simulink library "Pump_Additional"  (R2018b)
settings: Solver=ode45  StartTime=0.0  StopTime=10.0  RelTol=1e-3  EnableMultiTasking=on
undefined symbols (not defined in the file): DiameterLastPiece, DPConstant, DPLinear, DPQuadratic, ID, path_carnot, Pressure, Temperature
libraries: carnot x3
settings Model: Creator=Hafner  LastModifiedBy=drhf
settings DataIOCC: LimitDataPoints=on  SaveFormat=Array  SignalLoggingSaveFormat=ModelDataLogs
settings OptimizationCC: ExpressionDepthLimit=2147483647  LifeSpan=inf
settings DebuggingCC: UnderspecifiedInitializationDetection=Classic  MergeDetectMultiDrivingBlocksExec=none  SolverPrmCheckMsg=warning  FcnCallInpInsideContextMsg=warning  StateNameClashWarn=warning  SFUnexpectedBacktrackingDiag=warning  SFNoUnconditionalDefaultTransitionDiag=warning  SFExecutionAtInitializationDiag=none
settings HardwareCC: ProdBitPerPointer=32  ProdBitPerSizeT=32  ProdBitPerPtrDiffT=32  ProdLargestAtomicFloat=None  ProdIntDivRoundTo=Undefined  ProdEndianess=Unspecified  ProdWordSize=32  ProdHWDeviceType=32-bit Generic
settings ModelReferenceCC: PropagateSignalLabelsOutOfModel=off
settings SFSimCC: SimUseLocalCustomCode=off
settings RTWCC: RTWUseLocalCustomCode=off
settings CodeAppCC: StateflowObjectComments=on
settings GRTTargetCC: TargetLangStandard=C89/C90 (ANSI)  GeneratePreprocessorConditionals=Disable all  CombineOutputUpdateFcns=off  GRTInterface=on
settings ConfigComp: CovMetricSettings=dw  CovHtmlReporting=on  CovSaveCumulativeToWorkspaceVar=on  CovSaveSingleToWorkspaceVar=on  CovExternalEMLEnable=off

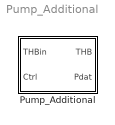
== system Pump_Additional ==
  Pump_Additional : Subsystem  mask(Pump Additional){Tini=20, PathName=fullfile(path_carnot('libsl'), 'Hydraulics', 'Pump_Main', 'parameter_set'), FileName='Pump6m.mat', userPath=off, userParam=off, a0=60000, a1=-43200, a2=0, dia=0.025, UA=1, mcp=4182, e0=50, e1=28.8, e2=-10.368}
      mask prompts: Tini "Ambient temperature for losses and initial temperture in °C"; PathName "Path"; FileName "Parameter set"; userPath "Edit path and name of parameter set"; userParam "User defined parameters"; a0 "a0: pump head in [Pa] (pressure increase at zero flow)"; a1 "a1: pump characteristic linear coefficient [Pa*s/kg]"; a2 "a2: pump characteristic quadratic coefficient [Pa*(s/kg)²]"; dia "Diameter at in- and outlet [m]"; UA "UA: thermal loss coefficient in W/K"; mcp "mcp: thermal capacity of the node in J/K"; e0 "e0: constant coefficient in W"; e1 "e1: linear coefficient in W*s/kg"; e2 "e2: quadratic coefficient in W*(s/kg)²"
      mask help:
      | This is an additional pump in a circuit. Every circuit must have exactly ONE 'Pump_Main'. It may have several 'Pump_Additional' blocks. The pump adds dp_pump to the pressure drop of the circuit dp_circuit:
      |     dp_circuit = c + l*mdot + q*(mdot)²
      |     dp_pump_ = a0*Ctrl + a1*mdot +a2*(mdot)²
      |     dp_total = dp_pump - dp_circuit
      |     p1 = system_pressure + (a0*Ctrl - c) + (a1 - l) * mdot + (a2-q)*(mdot)²
      | with
      |   Ctrl : Control signal input [0..1]
      | Note: Pump_Additional uses the parameters sets as Pump_Main.
      mask init:
      | % callback to set parameters of model
      | [ok, param] = CarnotCallbacks_PumpAdditional('SetParameters',gcbh,PathName,FileName);
      mask Help: web(fullfile(path_carnot('help'),'Pump_Main.html'),'-helpbrowser')
      mask TypeOptions Tini: ThermalNodeTHB/Tini
      mask Callback userPath: [ok, param] = CarnotCallbacks_PumpAdditional('UserEdit',gcbh);
      mask Callback userParam: [ok, param] = CarnotCallbacks_PumpAdditional('UserEdit',gcbh);
      mask TypeOptions a0: PumpHead/Gain
      mask TypeOptions a1: PumpLinear/Value
      mask TypeOptions a2: PumpQuadratic/Value
      mask TypeOptions dia: dia/Value
      mask TypeOptions UA: ThermalNodeTHB/UA
      mask TypeOptions mcp: ThermalNodeTHB/mcp
      mask TypeOptions e0: ElectricConsumptionPump/e0
      mask TypeOptions e1: ElectricConsumptionPump/e1
      mask TypeOptions e2: ElectricConsumptionPump/e2
      mask DialogControl ParameterGroupFile Prompt: Picking a parameter set
      mask DialogControl Control1 Prompt: Carnot public data
      mask DialogControl Control1 Callback: [ok, file] = CarnotCallbacks_PumpAdditional('GetFilename',gcbh,'public');
      mask DialogControl Control3 Prompt: Carnot internal data
      mask DialogControl Control3 Callback: [ok, file] = CarnotCallbacks_PumpAdditional('GetFilename',gcbh,'internal');
      mask DialogControl Control4 Prompt: Selected path
      mask DialogControl Control4 Callback: [ok, file] = CarnotCallbacks_PumpAdditional('GetFilename',gcbh,'selected');
      mask DialogControl PrameterGroupUser Prompt: Parameter Values
      mask DialogControl Container9 Prompt: Hydraulic
      mask DialogControl Container7 Prompt: Thermal
      mask DialogControl Control9 Prompt: Thermal node for temperature:  mcp * dTnode/dt = UA*(Tamb-Tnode) + mdot*cp_in*(Tin-Tnode)
      mask DialogControl Container12 Prompt: Electric
      mask DialogControl Control7 Prompt: Power consumption  Pel = e0 + e1*mdot + e2*mdot²
      mask DialogControl Control5 Prompt: Save in Carnot internal data
      mask DialogControl Control5 Callback: [ok, param] = CarnotCallbacks_PumpAdditional('SaveFilename',gcbh,'internal','B');
      mask DialogControl Control6 Prompt: Save in selected path
      mask DialogControl Control6 Callback: [ok, param] = CarnotCallbacks_PumpAdditional('SaveFilename',gcbh,'selected','B');
      mask Display:
      | % user defined picture file
      | picfile = fullfile(path_carnot('intlibsl'), ...
      |         'Hydraulics', 'Pump_Additional', 'PumpAdditional.jpg');
      | 
      | pic = false;
      | if ~BlockIsInCarnotLibrary    % if not located in library any more
      |     if exist(picfile,'file') % show internal picture if defined
      |         image(imread(picfile), [0.2, 0, 0.6, 1])
      |         set_param(gcb, 'BackgroundColor', 'White')
      |         pic = true;
      |     end
      | end
      | if ~pic    % show public picture
      |     set_param(gcb, 'BackgroundColor', 'green')
      |     plot(0,0,1,1,[40,70,40,30,30,40,60,70,70,60,40]/100, ...
      |         [70,50,30,40,60,70,70,60,40,30,30]/100)
      |     disp('add')
      | end

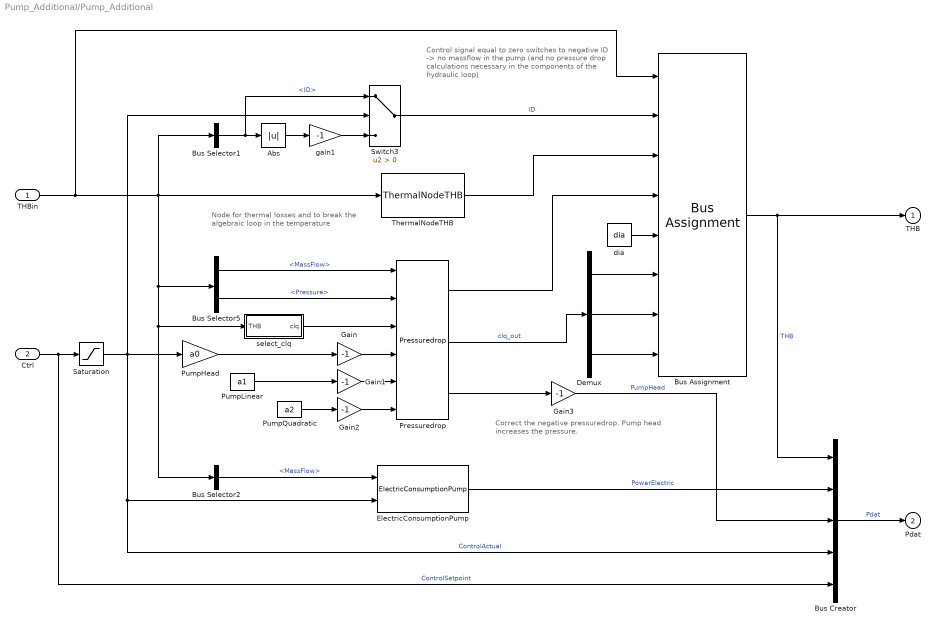
== system Pump_Additional/Pump_Additional ==
  note: Node for thermal losses and to break
      | the algebraic loop in the temperature
  note: Control signal equal to zero switches
      | to negative ID -> no massflow in the
      | pump (and no pressure drop calculations
      | necessary in the components of the
      | hydraulic loop)
  note: Correct the negative pressuredrop.
      | Pump head increases the pressure.
  THBin : Inport
  Ctrl : Inport  Port=2
  Abs : Abs
  Bus Assignment : BusAssignment  AssignedSignals=ID,Temperature,Pressure,DiameterLastPiece,DPConstant,DPLinear,DPQuadratic
  Bus Creator : BusCreator  Inputs=5
  Bus Selector1 : BusSelector  OutputSignals=ID
  Bus Selector2 : BusSelector  OutputSignals=MassFlow
  Bus Selector5 : BusSelector  OutputSignals=MassFlow,Pressure
  Demux : Demux  Outputs=3
  ElectricConsumptionPump : carnot/Basic/Hydraulics/ElectricConsumptionPump  e0=e0  e1=e1  e2=e2
      settings: SourceProductName=Carnot
  Gain{,1..3} (4 alike) : Gain  Gain=-1
  Pressuredrop : carnot/Basic/Pressure_Drop/Pressuredrop
      settings: SourceProductName=Carnot
  PumpHead : Gain  Gain=a0
  PumpLinear : Constant  Value=a1
  PumpQuadratic : Constant  Value=a2
  Saturation : Saturate  UpperLimit=1  LowerLimit=0
  Switch3 : Switch  Criteria=u2 > Threshold  SaturateOnIntegerOverflow=on  InputSameDT=on
  ThermalNodeTHB : carnot/Basic/Thermal_Models/ThermalNodeTHB  UA=UA  mcp=mcp  Tini=Tini
      settings: SourceProductName=Carnot
  dia : Constant  Value=dia
  gain1 : Gain  Gain=-1  SaturateOnIntegerOverflow=on  OutDataTypeStr=Inherit: Same as input  ParamDataTypeStr=Inherit: Same as input
  select_clq : Subsystem
  THB : Outport
  Pdat : Outport  Port=2
  wires:
  Gain2/1 -> Pressuredrop/6
  Gain1/1 -> Pressuredrop/5
  Gain/1 -> Pressuredrop/4
  Bus Selector5/2 -> Pressuredrop/2  "<Pressure>"
  select_clq/1(clq) -> Pressuredrop/3
  ThermalNodeTHB/1 -> Bus Assignment/3
  Demux/3 -> Bus Assignment/8
  Demux/2 -> Bus Assignment/7
  Demux/1 -> Bus Assignment/6
  PumpQuadratic/1 -> Gain2/1
  PumpLinear/1 -> Gain1/1
  PumpHead/1 -> Gain/1
  THBin/1 -> Bus Assignment/1, ThermalNodeTHB/1, Bus Selector1/1, Bus Selector5/1, Bus Selector2/1, select_clq/1(THB)
  dia/1 -> Bus Assignment/5
  Bus Selector5/1 -> Pressuredrop/1  "<MassFlow>"
  Switch3/1 -> Bus Assignment/2  "ID"
  gain1/1 -> Switch3/3
  Abs/1 -> gain1/1
  Bus Selector1/1 -> Abs/1, Switch3/1  "<ID>"
  Ctrl/1 -> Bus Creator/5, Saturation/1  "ControlSetpoint"
  ElectricConsumptionPump/1 -> Bus Creator/2  "PowerElectric"
  Bus Creator/1 -> Pdat/1  "Pdat"
  Bus Selector2/1 -> ElectricConsumptionPump/1  "<MassFlow>"
  Bus Assignment/1 -> Bus Creator/1, THB/1  "THB"
  Pressuredrop/3 -> Gain3/1
  Pressuredrop/2 -> Demux/1  "clq_out"
  Pressuredrop/1 -> Bus Assignment/4
  Gain3/1 -> Bus Creator/3  "PumpHead"
  Saturation/1 -> ElectricConsumptionPump/2, Bus Creator/4, PumpHead/1, Switch3/2  "ControlActual"

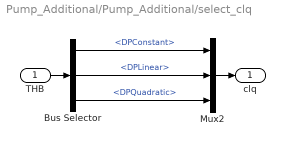
== system Pump_Additional/Pump_Additional/select_clq ==
  THB : Inport
  Bus Selector : BusSelector  OutputSignals=DPConstant,DPLinear,DPQuadratic
  Mux2 : Mux  Inputs=3
  clq : Outport
  wires:
  Bus Selector/3 -> Mux2/3  "<DPQuadratic>"
  Bus Selector/2 -> Mux2/2  "<DPLinear>"
  Bus Selector/1 -> Mux2/1  "<DPConstant>"
  THB/1 -> Bus Selector/1
  Mux2/1 -> clq/1
